simulink model "affineManeuver"  (R2021b)
settings: Solver=ode4  StartTime=0.0  StopTime=10.0  FixedStep=0.01  MaxStep=0.02  RelTol=1e-3  EnableMultiTasking=on
values from neighbouring files (symbols this model uses):
  dim = 2    [main.m]
  nodenum = size(P,1)    [main.m]
  stepsize = 0.005    [main.m]
  v_init = zeros(dim*nodenum,1)    [main.m]
  x_init = p+[0 0 0 0 0 0 1 1 0 1 -1 1 -2 -1]'    [main.m]
settings Model: Creator=Shiyu Zhao  LastModifiedBy=asachd11
settings SolverCC: AlgebraicLoopSolver=TrustRegion
settings DataIOCC: LimitDataPoints=on  SaveFormat=Array  SignalLoggingSaveFormat=ModelDataLogs  ReturnWorkspaceOutputs=off
settings OptimizationCC: ExpressionDepthLimit=2147483647  LifeSpan=inf
settings DebuggingCC: UnderspecifiedInitializationDetection=Classic  MergeDetectMultiDrivingBlocksExec=none  SolverPrmCheckMsg=warning  FcnCallInpInsideContextMsg=warning  StateNameClashWarn=warning  SFUnexpectedBacktrackingDiag=warning  SFNoUnconditionalDefaultTransitionDiag=warning  SFExecutionAtInitializationDiag=none  SFMachineParentedDataDiag=warning  ArithmeticOperatorsInVariantConditions=warning
settings HardwareCC: ProdBitPerPointer=32  ProdBitPerSizeT=32  ProdBitPerPtrDiffT=32  ProdLargestAtomicFloat=None  ProdIntDivRoundTo=Undefined  ProdEndianess=Unspecified  ProdWordSize=32  ProdHWDeviceType=32-bit Generic
settings ModelReferenceCC: PropagateSignalLabelsOutOfModel=off
settings SFSimCC: SimUseLocalCustomCode=off  CustomCodeUndefinedFunction=UseInterfaceOnly
settings RTWCC: RTWUseLocalCustomCode=off
settings CodeAppCC: StateflowObjectComments=on
settings GRTTargetCC: TargetLangStandard=C89/C90 (ANSI)  CombineOutputUpdateFcns=off  GRTInterface=on
settings ConfigComp: CovMetricSettings=dw  CovSaveCumulativeToWorkspaceVar=on  CovSaveSingleToWorkspaceVar=on  CovExternalEMLEnable=off

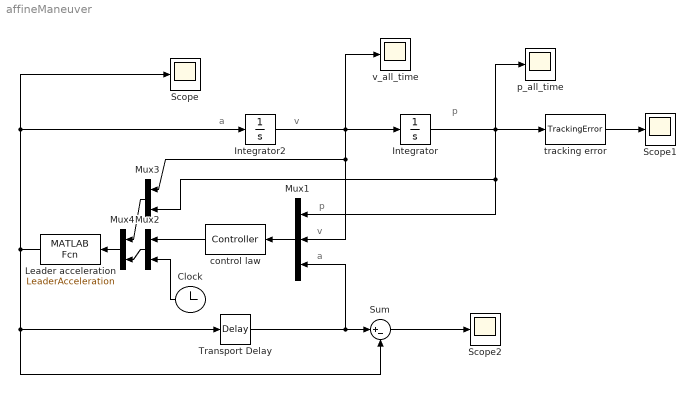
== system affineManeuver ==
  note: a
  note: p
  note: v
  note: p
  note: v
  note: a
  Clock : Clock
  Integrator : Integrator  InitialCondition=x_init
  Integrator2 : Integrator  InitialCondition=v_init
  Leader acceleration : MATLABFcn  MATLABFcn=LeaderAcceleration
  Mux1 : Mux  Inputs=3
  Mux2 : Mux  Inputs=2
  Mux3 : Mux  Inputs=2
  Mux4 : Mux  Inputs=2
  Scope : Scope
  Scope1 : Scope
  Scope2 : Scope
  Sum : Sum  Inputs=|+-
  Transport Delay : TransportDelay  DelayTime=stepsize  InitialOutput=zeros(dim*nodenum,1)
  control law : MATLABFcn  MATLABFcn=Controller
  p_all_time : Scope
  tracking error : MATLABFcn  MATLABFcn=TrackingError
  v_all_time : Scope
  wires:
  tracking error/1 -> Scope1/1
  Mux1/1 -> control law/1
  Integrator/1 -> tracking error/1, p_all_time/1, Mux1/1, Mux3/2
  Integrator2/1 -> Integrator/1, v_all_time/1, Mux1/2, Mux3/1
  control law/1 -> Mux2/1
  Clock/1 -> Mux2/2
  Leader acceleration/1 -> Integrator2/1, Scope/1, Sum/2, Transport Delay/1
  Transport Delay/1 -> Mux1/3, Sum/1
  Sum/1 -> Scope2/1
  Mux3/1 -> Mux4/1
  Mux2/1 -> Mux4/2
  Mux4/1 -> Leader acceleration/1
